simulink subsystem "Encoder_A_Metros"  (R2024b)
settings: Solver=VariableStepAuto  StartTime=0.0  StopTime=10.0  RelTol=1e-3
libraries: arduinosensorlib x2
settings Model: Creator=Chenfu  LastModifiedBy=lucia

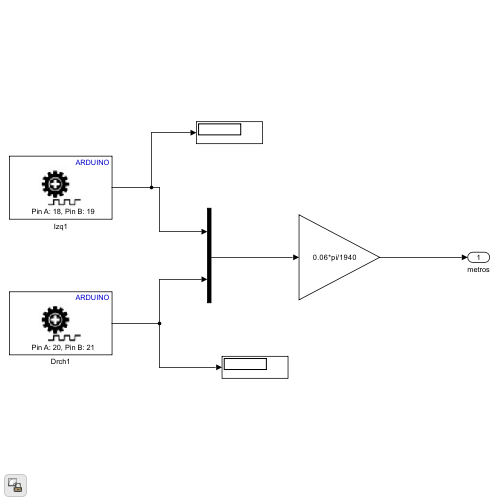
[thumbnail: Simulink's stored preview of the top-level diagram]
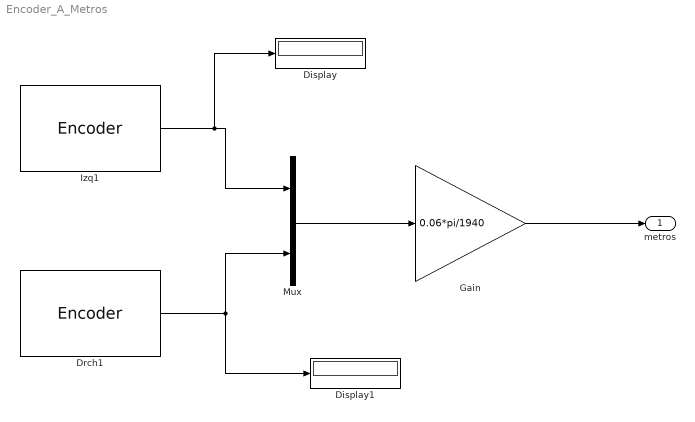
== system Encoder_A_Metros ==
  Display : Display
  Display1 : Display
  Drch1 : arduinosensorlib/Encoder  InputA=20  InputB=21  Mode=No reset  SampleTime=-1
  Gain : Gain  Gain=0.06*pi/1940  OutDataTypeStr=double
  Izq1 : arduinosensorlib/Encoder  InputA=18  InputB=19  Mode=No reset  SampleTime=-1
  Mux : Mux  Inputs=2
  metros : Outport
  wires:
  Mux/1 -> Gain/1
  Gain/1 -> metros/1
  Izq1/1 -> Mux/1, Display/1
  Drch1/1 -> Display1/1, Mux/2
